simulink model "practice2"  (R2023a)
settings: Solver=VariableStepAuto  StartTime=0.0  StopTime=10.0  RelTol=1e-3
settings Model: Creator=fxin  LastModifiedBy=fxin

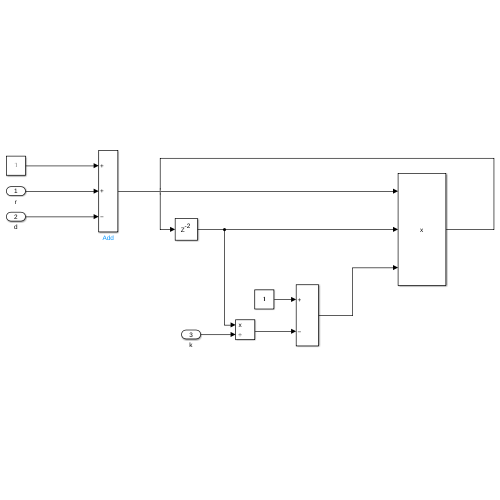
[thumbnail: Simulink's stored preview of the top-level diagram]
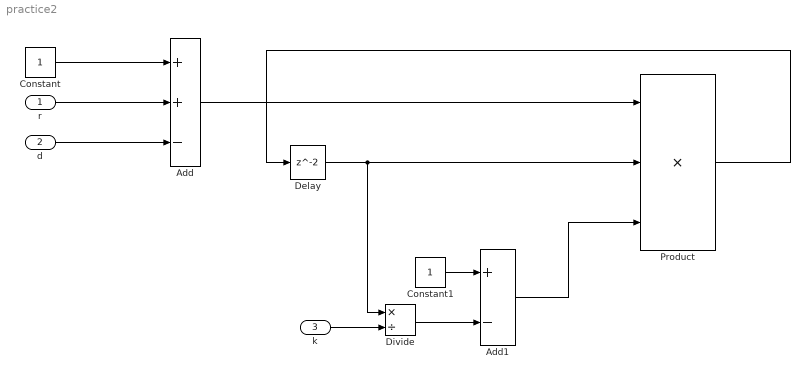
== system practice2 ==
  r : Inport
  d : Inport  Port=2
  k : Inport  Port=3
  Add : Sum  Inputs=++-
  Add1 : Sum  Inputs=+-
  Constant : Constant
  Constant1 : Constant
  Delay : Delay
  Divide : Product  Inputs=*/
  Product : Product  Inputs=3
  wires:
  Constant/1 -> Add/1
  r/1 -> Add/2
  d/1 -> Add/3
  Add/1 -> Product/1
  Delay/1 -> Divide/1, Product/2
  Constant1/1 -> Add1/1
  Divide/1 -> Add1/2
  Add1/1 -> Product/3
  Product/1 -> Delay/1
  k/1 -> Divide/2
